simulink model "raise_cosine"  (Simulink 7.9)
settings: Solver=FixedStepDiscrete  SolverMode=SingleTasking  StartTime=0.0  StopTime=100e-3  FixedStep=1/100000  RelTol=1e-3  AbsTol=1e-6
libraries: dspsrcs4 x2, commfilt2 x1
settings Model: Creator=amoura  LastModifiedBy=amoura_2
settings DataIOCC: LimitDataPoints=off  SignalLoggingName=sigsOut
settings OptimizationCC: BooleanDataType=off  InitFltsAndDblsToZero=on
settings DebuggingCC: SaveWithParameterizedLinksMsg=none  SignalResolutionControl=TryResolveAllWithWarning  SolverPrmCheckMsg=none  MultiTaskDSMMsg=warning  MultiTaskCondExecSysMsg=none  FcnCallInpInsideContextMsg=Use local settings  StrictBusMsg=None
settings HardwareCC: TargetUnknown=on
settings RTWCC: TemplateMakefile=grt_unix.tmf  IncludeERTFirstTime=on
settings GRTTargetCC: TargetFcnLib=ansi_tfl_tmw.mat  ModelReferenceCompliant=off  CombineOutputUpdateFcns=off  MatFileLogging=off  GRTInterface=on

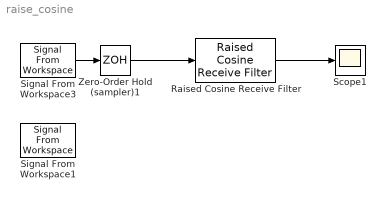
== system raise_cosine ==
  Raised Cosine Receive Filter : commfilt2/Raised Cosine Receive Filter  filtType=Normal  N=100  D=6  R=0  sampMode=Mute  saveAsFlag=0  rateMode=None  downFactor=8  downOffset=0  framing=Allow multirate processing  InputProcessing=Inherited (this choice will be removed - see release notes)  checkGain=User-specified  filterGain=1/100  checkCoeff=off  variableName=rcRxFilt  launchFVT=off  roundingMode=Floor  overflowMode=off
  Scope1 : Scope
      settings: TickLabels=on
  Signal From Workspace1 : dspsrcs4/Signal From Workspace  X=randi([0 1],1000,1)  Ts=1/1000  nsamps=1  OutputAfterFinalValue=Cyclic repetition  ignoreOrWarnInputAndFrameLengths=off
  Signal From Workspace3 : dspsrcs4/Signal From Workspace  X=[0 0 0 0 0 1 0 0 0 0 0 ]  Ts=1/1000  nsamps=1  OutputAfterFinalValue=Cyclic repetition  ignoreOrWarnInputAndFrameLengths=off
  Zero-Order Hold (sampler)1 : ZeroOrderHold  SampleTime=1/100000
  wires:
  Signal From Workspace3/1 -> Zero-Order Hold (sampler)1/1
  Raised Cosine Receive Filter/1 -> Scope1/1
  Zero-Order Hold (sampler)1/1 -> Raised Cosine Receive Filter/1
